simulink model "starmac_system"  (Simulink 7.1)
settings: Solver=ode45  StartTime=0.0  StopTime=30  FixedStep=.001  MaxStep=.01  RelTol=1e-4
undefined symbols (not defined in the file or in its folder): DiscIntNeverNeededParam, ToverTh
libraries: simulink x12, aero_sim_lib x1
settings Model: Creator=Administrator  LastModifiedBy=Administrator

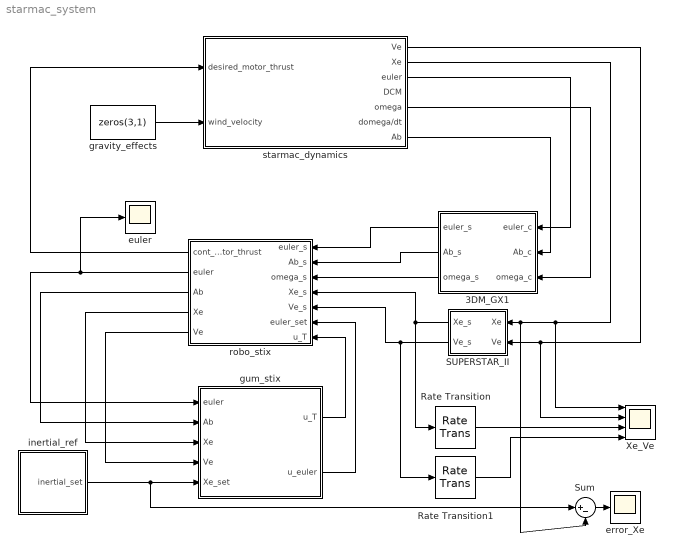
== system starmac_system ==
  3DM_GX1 : Subsystem  Orientation=left  mask{a_g_s=7000, g_max=5, g_g_s=8500, omega_max=300, Ts=.01}
      mask prompts: a_g_s "AccelGainScale:"; g_max "Max G (1 G = 9.81 m/s^2):"; g_g_s "GyroGainScale:"; omega_max "Mav Angular Velocity (deg/sec):"; Ts "Sample Rate (seconds):"
  Rate Transition : RateTransition
  Rate Transition1 : RateTransition
  SUPERSTAR_II : Subsystem  Orientation=left  mask{Ts=.2}
      mask prompts: Ts "Sample Rate (seconds):"
  Sum : Sum  Inputs=|+-  OutDataType=sfix(16)  OutScaling=2^0
  Xe_Ve : Scope  NumInputPorts=4
      settings: YMin=-5~-5~-5~-5  YMax=5~5~5~5
  error_Xe : Scope
      settings: SaveName=ScopeData4
  euler : Scope
  gravity_effects : Constant  Value=zeros(3,1)  OutDataType=sfix(16)  OutScaling=2^0
  gum_stix : Subsystem
  inertial_ref : Subsystem
  robo_stix : Subsystem  Orientation=left
  starmac_dynamics : Subsystem  AncestorBlock=aero_sim_lib/starmac_dynamics  mask{M=1.8263, tau_motor=0.1, b=0.1, select_sub=Select Subsystem}
      mask prompts: M "UAV Mass (kg) [M]:"; tau_motor "Motor Time constant (s)[tau_motor]:"; b "Viscus Drag Coef. (N-s/m)[b]:"; select_sub "Select a model Subsystem:"
      mask StyleString: edit,edit,edit,popup(Select Subsystem|M:starmac_motor_dynamics|B:starmac_blade_flapping_effects|6:6DOF_Euler_Angles)
      mask CallbackString:
      | |||gcb_d=gcb;
      | mask_str = get_param(gcb_d, 'MaskValues');
      | if strcmp(mask_str{4}(1),'M')
      |     open_system([gcb_d '/starmac_motor_dynamics'],'mask');
      | elseif strcmp(mask_str{4}(1),'B')
      |     open_system([gcb_d '/starmac_blade_flapping_effects'],'mask');
      | elseif strcmp(mask_str{4}(1),'6')
      |     open_system([gcb_d '/6DOF_Euler_Angles'],'mask');
      | else
      |     return
      | end
      | set_param(gcb_d,'select_sub','Select Subsystem');
  wires:
  robo_stix/1(cont_motor_thrust) -> starmac_dynamics/1(desired_motor_thrust)
  starmac_dynamics/3(euler) -> 3DM_GX1/1(euler_c)
  starmac_dynamics/7(Ab) -> 3DM_GX1/2(Ab_c)
  starmac_dynamics/5(omega) -> 3DM_GX1/3(omega_c)
  3DM_GX1/1(euler_s) -> robo_stix/1(euler_s)
  3DM_GX1/2(Ab_s) -> robo_stix/2(Ab_s)
  3DM_GX1/3(omega_s) -> robo_stix/3(omega_s)
  robo_stix/2(euler) -> gum_stix/1(euler), euler/1
  robo_stix/4(Xe) -> gum_stix/3(Xe)
  robo_stix/5(Ve) -> gum_stix/4(Ve)
  gum_stix/1(u_T) -> robo_stix/7(u_T)
  gum_stix/2(u_euler) -> robo_stix/6(euler_set)
  robo_stix/3(Ab) -> gum_stix/2(Ab)
  SUPERSTAR_II/1(Xe_s) -> robo_stix/4(Xe_s), Rate Transition/1
  SUPERSTAR_II/2(Ve_s) -> robo_stix/5(Ve_s), Rate Transition1/1
  starmac_dynamics/2(Xe) -> Xe_Ve/1, SUPERSTAR_II/1(Xe), Sum/2
  starmac_dynamics/1(Ve) -> SUPERSTAR_II/2(Ve), Xe_Ve/2
  inertial_ref/1(inertial_set) -> gum_stix/5(Xe_set), Sum/1
  gravity_effects/1 -> starmac_dynamics/2(wind_velocity)
  Sum/1 -> error_Xe/1
  Rate Transition/1 -> Xe_Ve/3
  Rate Transition1/1 -> Xe_Ve/4

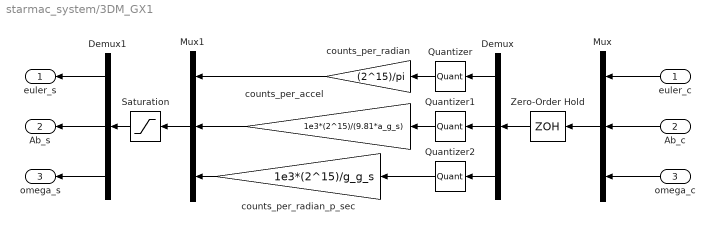
== system starmac_system/3DM_GX1 ==
  euler_c : Inport  Orientation=left
  Ab_c : Inport  Orientation=left  Port=2
  omega_c : Inport  Orientation=left  Port=3
  Demux : Demux  Orientation=left  Outputs=[3 3 3]
  Demux1 : Demux  Orientation=left  Outputs=[3 3 3]
  Mux : Mux  Orientation=left  Inputs=[3 3 3]
  Mux1 : Mux  Orientation=left  Inputs=3
  Quantizer : Quantizer  Orientation=left  QuantizationInterval=pi/(2^15)*ones(3,1)
  Quantizer1 : Quantizer  Orientation=left  QuantizationInterval=g_max*9.81/(2^15)*ones(3,1)
  Quantizer2 : Quantizer  Orientation=left  QuantizationInterval=(pi*omega_max/180)/(2^15)*ones(3,1)
  Saturation : Saturate  Orientation=left  UpperLimit=((2^15)-1)*ones(3*3,1)  LowerLimit=-(2^15)*ones(3*3,1)  OutDataType=sfix(16)  OutScaling=2^0
  Zero-Order Hold : ZeroOrderHold  Orientation=left  SampleTime=Ts
  counts_per_accel : Gain  Orientation=left  Gain=1e3*(2^15)/(9.81*a_g_s)  ParameterDataType=sfix(16)  ParameterScaling=2^0  OutDataType=sfix(16)  OutScaling=2^0
  counts_per_radian : Gain  Orientation=left  Gain=(2^15)/pi  ParameterDataType=sfix(16)  ParameterScaling=2^0  OutDataType=sfix(16)  OutScaling=2^0
  counts_per_radian_p_sec : Gain  Orientation=left  Gain=1e3*(2^15)/g_g_s  ParameterDataType=sfix(16)  ParameterScaling=2^0  OutDataType=sfix(16)  OutScaling=2^0
  euler_s : Outport  Orientation=left
  Ab_s : Outport  Orientation=left  Port=2
  omega_s : Outport  Orientation=left  Port=3
  wires:
  Mux/1 -> Zero-Order Hold/1
  euler_c/1 -> Mux/1
  Ab_c/1 -> Mux/2
  omega_c/1 -> Mux/3
  Zero-Order Hold/1 -> Demux/1
  Demux/1 -> Quantizer/1
  Demux/2 -> Quantizer1/1
  Quantizer/1 -> counts_per_radian/1
  Quantizer1/1 -> counts_per_accel/1
  counts_per_accel/1 -> Mux1/2
  counts_per_radian/1 -> Mux1/1
  Demux/3 -> Quantizer2/1
  counts_per_radian_p_sec/1 -> Mux1/3
  Quantizer2/1 -> counts_per_radian_p_sec/1
  Mux1/1 -> Saturation/1
  Saturation/1 -> Demux1/1
  Demux1/1 -> euler_s/1
  Demux1/2 -> Ab_s/1
  Demux1/3 -> omega_s/1

== system starmac_system/SUPERSTAR_II ==
  Xe : Inport  Orientation=left
  Ve : Inport  Orientation=left  Port=2
  Demux : Demux  Orientation=left  Outputs=[3 3]
  Mux : Mux  Orientation=left  Inputs=[3 3]
  ZOH : ZeroOrderHold  Orientation=left  SampleTime=Ts
  Xe_s : Outport  Orientation=left
  Ve_s : Outport  Orientation=left  Port=2
  wires:
  ZOH/1 -> Demux/1
  Ve/1 -> Mux/2
  Xe/1 -> Mux/1
  Mux/1 -> ZOH/1
  Demux/1 -> Xe_s/1
  Demux/2 -> Ve_s/1

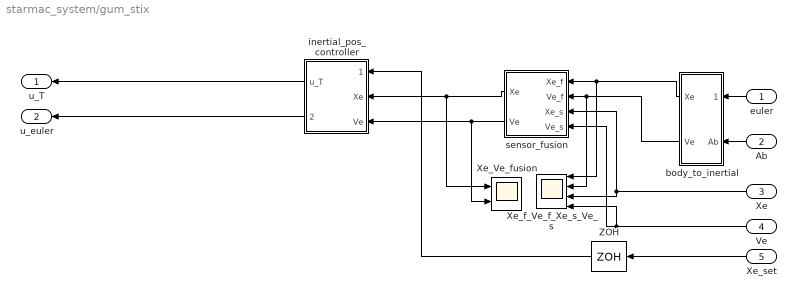
== system starmac_system/gum_stix ==
  euler : Inport  Orientation=left
  Ab : Inport  Orientation=left  Port=2
  Xe : Inport  Orientation=left  Port=3
  Ve : Inport  Orientation=left  Port=4
  Xe_set : Inport  Orientation=left  Port=5
  Xe_Ve_fusion : Scope  NumInputPorts=2
      settings: YMin=-10~-5  YMax=10~5  SaveName=ScopeData2
  Xe_f_Ve_f_Xe_s_Ve_s : Scope  NumInputPorts=4
      settings: YMin=-5~-5~-5~-5  YMax=5~5~5~5  SaveName=ScopeData3
  ZOH : ZeroOrderHold  Orientation=left  SampleTime=.01
  body_to_inertial : Subsystem  Orientation=left
  inertial_pos_controller : Subsystem  Orientation=left  mask{Ts=.01, M=1.8263, K=7.5, K_Ve=2.5}
      mask prompts: Ts "Enter Sample Time [Ts] (seconds):"; M "Enter Mass of UAV [M] (kg):"; K "Enter Loop Gain [K]:"; K_Ve "Enter Velocity Damping Gain [K_Ve]:"
  sensor_fusion : Subsystem  Orientation=left
  u_T : Outport  Orientation=left
  u_euler : Outport  Orientation=left  Port=2
  wires:
  Xe_set/1 -> ZOH/1
  inertial_pos_controller/1(u_T) -> u_T/1
  inertial_pos_controller/2(u_euler) -> u_euler/1
  euler/1 -> body_to_inertial/1(euler)
  Ab/1 -> body_to_inertial/2(Ab)
  sensor_fusion/1(Xe) -> inertial_pos_controller/2(Xe), Xe_Ve_fusion/1
  sensor_fusion/2(Ve) -> inertial_pos_controller/3(Ve), Xe_Ve_fusion/2
  body_to_inertial/1(Xe) -> sensor_fusion/1(Xe_f), Xe_f_Ve_f_Xe_s_Ve_s/1
  body_to_inertial/2(Ve) -> sensor_fusion/2(Ve_f), Xe_f_Ve_f_Xe_s_Ve_s/2
  Xe/1 -> sensor_fusion/3(Xe_s), Xe_f_Ve_f_Xe_s_Ve_s/3
  Ve/1 -> sensor_fusion/4(Ve_s), Xe_f_Ve_f_Xe_s_Ve_s/4
  ZOH/1 -> inertial_pos_controller/1(Xe_set)

== system starmac_system/inertial_ref ==
  Signal Generator : SignalGenerator  Amplitude=20*[1 -1 .5]  Frequency=.5*.0625*ones(3,1)
  inertial_set : Outport
  wires:
  Signal Generator/1 -> inertial_set/1

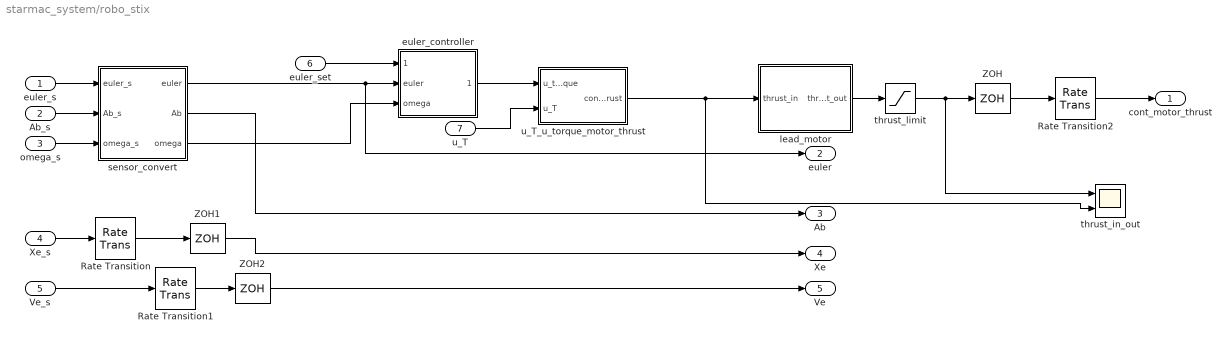
== system starmac_system/robo_stix ==
  euler_s : Inport
  Ab_s : Inport  Port=2
  omega_s : Inport  Port=3
  Xe_s : Inport  Port=4
  Ve_s : Inport  Port=5
  euler_set : Inport  Port=6
  u_T : Inport  Port=7
  Rate Transition : RateTransition
  Rate Transition1 : RateTransition
  Rate Transition2 : RateTransition
  ZOH : ZeroOrderHold  SampleTime=.01
  ZOH1 : ZeroOrderHold  SampleTime=.01
  ZOH2 : ZeroOrderHold  SampleTime=.01
  euler_controller : Subsystem  mask{K=1, K_e=7.5, K_o=.65}
      mask prompts: K "Loop Gain [K]:"; K_e "Euler Gain [K_e]:"; K_o "Omega Gain [K_o]:"
  lead_motor : Subsystem  mask{tau_motor=.1, t_s=.01}
      mask init:
      | a=1/tau_motor;
      | b=pi/t_s;
      | T=t_s;
      | num1=b*(1-exp(-b*T))+a*(b*T-1+exp(-b*T));
      | num2=-b*(1-exp(-b*T))+a*(1-exp(-b*T)-b*T*exp(-b*T));
      | den1=a*b;
      | den2=-a*b*exp(-b*T);
      | num=(b/a)*[num1 num2];
      | den=[den1 den2];
      | Hz=tf(num,den,T);
      | [y,t]=step(Hz);
      | num=(1/y(length(y)))*num;
      | %Hz=(1/y(length(y)))*Hz
      | %bode(Hz);
  sensor_convert : Subsystem  mask{a_g_s=7000, g_g_s=8500}
      mask prompts: a_g_s "AccelGainScale[a_g_s]:"; g_g_s "GyroGainScale[g_g_s]:"
  thrust_in_out : Scope  NumInputPorts=2
      settings: YMin=-5~-5  YMax=5~5  SaveName=ScopeData5
  thrust_limit : Saturate  UpperLimit=10*ones(1,4)  LowerLimit=0*ones(1,4)  OutDataType=sfix(16)  OutScaling=2^0
  u_T_u_torque_motor_thrust : Subsystem  mask{dx=.3048, K_torque=.47}
      mask prompts: dx "X distance of motor from CG [dx](meters):"; K_torque "Ktorque [K_torque]:"
      mask init:
      | M=[0 -dx 0 dx;
      |    dx 0 -dx 0;
      |    -K_torque K_torque -K_torque K_torque;
      |    1 1 1 1];
      | Mi=inv(M);
  cont_motor_thrust : Outport
  euler : Outport  Port=2
  Ab : Outport  Port=3
  Xe : Outport  Port=4
  Ve : Outport  Port=5
  wires:
  euler_s/1 -> sensor_convert/1(euler_s)
  ZOH/1 -> Rate Transition2/1
  Ab_s/1 -> sensor_convert/2(Ab_s)
  omega_s/1 -> sensor_convert/3(omega_s)
  sensor_convert/1(euler) -> euler_controller/2(euler), euler/1
  euler_set/1 -> euler_controller/1(euler_set)
  sensor_convert/3(omega) -> euler_controller/3(omega)
  u_T/1 -> u_T_u_torque_motor_thrust/2(u_T)
  Xe_s/1 -> Rate Transition/1
  Ve_s/1 -> Rate Transition1/1
  euler_controller/1(u_torque) -> u_T_u_torque_motor_thrust/1(u_torque)
  sensor_convert/2(Ab) -> Ab/1
  ZOH1/1 -> Xe/1
  ZOH2/1 -> Ve/1
  Rate Transition/1 -> ZOH1/1
  Rate Transition1/1 -> ZOH2/1
  Rate Transition2/1 -> cont_motor_thrust/1
  u_T_u_torque_motor_thrust/1(cont_motor_thrust) -> lead_motor/1(thrust_in), thrust_in_out/2
  thrust_limit/1 -> ZOH/1, thrust_in_out/1
  lead_motor/1(thrust_out) -> thrust_limit/1

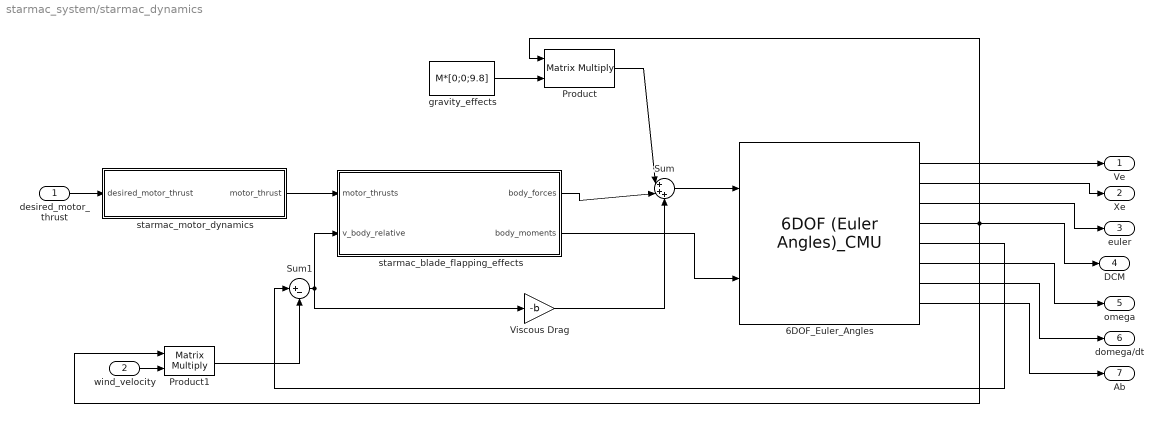
== system starmac_system/starmac_dynamics ==
  desired_motor_thrust : Inport  OutDataType=sfix(16)  OutScaling=2^0
  wind_velocity : Inport  Port=2  OutDataType=sfix(16)  OutScaling=2^0
  6DOF_Euler_Angles : aero_sim_lib/6DOF (Euler Angles)_CMU  SystemSampleTime=-1  XYZe_0=[0.1;0.2;0]  Vb_0=[0;0;0]  euler_0=[0;0;0]  omega_0=[0;0;0]  M=M  I=diag([0.02759 0.02771 0.04806])
  Product : Product  Multiplication=Matrix(*)  OutDataType=sfix(16)  OutScaling=2^0  RndMeth=Zero
  Product1 : Product  Multiplication=Matrix(*)  OutDataType=sfix(16)  OutScaling=2^0  RndMeth=Zero
  Sum : Sum  Inputs=|+++  OutDataType=sfix(16)  OutScaling=2^0
  Sum1 : Sum  Inputs=|+-  OutDataType=sfix(16)  OutScaling=2^0
  Viscous Drag : Gain  Gain=-b  ParameterDataType=sfix(16)  ParameterScaling=2^0  OutDataType=sfix(16)  OutScaling=2^0
  gravity_effects : Constant  Value=M*[0;0;9.8]  OutDataType=sfix(16)  OutScaling=2^0
  starmac_blade_flapping_effects : Subsystem  AncestorBlock=aero_sim_lib/starmac_blade_flapping_effects  mask{select_sub=Select Subsystem}
      mask prompts: select_sub "Select Subsystem:"
      mask help:
      | Allows user to set parameters of various subsystems
      | within the Blade Flapping Effects Model
      mask Help:
      | Select a Subsystem To Set Various
      | Sub System Parameters
      mask StyleString: popup(Select Subsystem|V:starmac_vertical_effect_dynamics|B:starmac_body_moments|F:starmac_flapping_dynamics)
      mask CallbackString:
      | gcb_c=gcb;
      | mask_str = get_param(gcb_c, 'MaskValues');
      | if strcmp(mask_str{1}(1),'V')
      |     open_system([gcb_c '/starmac_vertical_effect_dynamics'],'mask');
      | elseif strcmp(mask_str{1}(1),'B')
      |     open_system([gcb_c '/starmac_body_moments'],'mask');
      | elseif strcmp(mask_str{1}(1),'F')
      |     open_system([gcb_c '/starmac_flapping_dynamics'],'mask');
      | else
      |     return
      | end
      | set_param(gcb_c,'select_sub','Select Subsystem');
  starmac_motor_dynamics : Subsystem  AncestorBlock=aero_sim_lib/starmac_motor_dynamics  mask{tau_motor=tau_motor, T_nom=M*9.8/4, thrust_max=9.8, thrust_min=0, motor_lag_enable=on, motor_variance=(.05*9.8/4)^2, Ts=.01}
      mask prompts: tau_motor "tau_motor (seconds):"; T_nom "nominal thrust (N):"; thrust_max "maximum thrust (N):"; thrust_min "minimum thrust (N):"; motor_lag_enable "Motor Lag Enabled:"; motor_variance "Motor Variance [motor_variance]:"; Ts "Motor Update Rate (seconds):"
  Ve : Outport  OutDataType=sfix(16)  OutScaling=2^0
  Xe : Outport  Port=2  OutDataType=sfix(16)  OutScaling=2^0
  euler : Outport  Port=3  OutDataType=sfix(16)  OutScaling=2^0
  DCM : Outport  Port=4  OutDataType=sfix(16)  OutScaling=2^0
  omega : Outport  Port=5  OutDataType=sfix(16)  OutScaling=2^0
  domega/dt : Outport  Port=6  OutDataType=sfix(16)  OutScaling=2^0
  Ab : Outport  Port=7  OutDataType=sfix(16)  OutScaling=2^0
  wires:
  6DOF_Euler_Angles/8 -> Ab/1
  6DOF_Euler_Angles/7 -> domega/dt/1
  6DOF_Euler_Angles/6 -> omega/1
  6DOF_Euler_Angles/3 -> euler/1
  6DOF_Euler_Angles/2 -> Xe/1
  6DOF_Euler_Angles/1 -> Ve/1
  starmac_motor_dynamics/1(motor_thrust) -> starmac_blade_flapping_effects/1(motor_thrusts)
  Product/1 -> Sum/1
  Sum/1 -> 6DOF_Euler_Angles/1
  6DOF_Euler_Angles/4 -> DCM/1, Product/1, Product1/1
  gravity_effects/1 -> Product/2
  Sum1/1 -> starmac_blade_flapping_effects/2(v_body_relative), Viscous Drag/1
  Product1/1 -> Sum1/2
  6DOF_Euler_Angles/5 -> Sum1/1
  Viscous Drag/1 -> Sum/3
  starmac_blade_flapping_effects/2(body_moments) -> 6DOF_Euler_Angles/2
  starmac_blade_flapping_effects/1(body_forces) -> Sum/2
  desired_motor_thrust/1 -> starmac_motor_dynamics/1(desired_motor_thrust)
  wind_velocity/1 -> Product1/2

== system starmac_system/gum_stix/body_to_inertial ==
  euler : Inport  Orientation=left
  Ab : Inport  Orientation=left  Port=2
  Ab_to_Ae : Stateflow chart  Orientation=left
  Mux : Mux  Orientation=left  Inputs=[3 3]
  inertial_vel_and pos_est : Subsystem  Orientation=left  mask{Ts=.01}
      mask prompts: Ts "Sample Time [Ts] (seconds):"
  Xe : Outport  Orientation=left
  Ve : Outport  Orientation=left  Port=2
  wires:
  euler/1 -> Mux/1
  Ab/1 -> Mux/2
  inertial_vel_and pos_est/2(Xb) -> Xe/1
  Ab_to_Ae/1(y) -> inertial_vel_and pos_est/1(Ab)
  inertial_vel_and pos_est/1(Vb) -> Ve/1
  Mux/1 -> Ab_to_Ae/1(u)

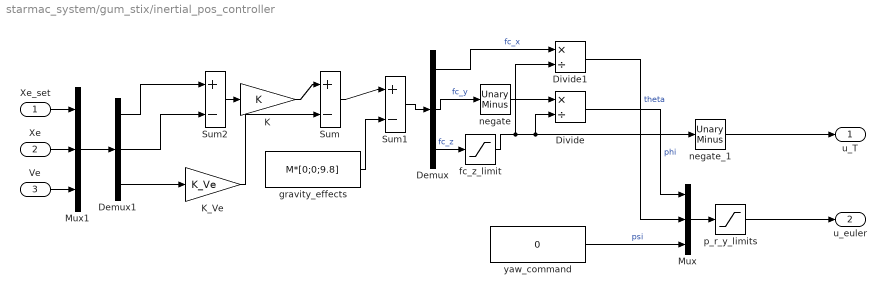
== system starmac_system/gum_stix/inertial_pos_controller ==
  Xe_set : Inport
  Xe : Inport  Port=2
  Ve : Inport  Port=3
  Demux : Demux  Outputs=[1 1 1]
  Demux1 : Demux  Outputs=[3 3 3]
  Divide : Product  Inputs=*/  OutDataType=sfix(16)  OutScaling=2^-10
  Divide1 : Product  Inputs=*/  OutDataType=sfix(16)  OutScaling=2^-10
  K : Gain  Gain=K  ParameterDataType=sfix(16)  ParameterScaling=2^0  OutDataType=sfix(16)  OutScaling=2^0
  K_Ve : Gain  Gain=K_Ve  ParameterDataType=sfix(16)  ParameterScaling=2^0  OutDataType=sfix(16)  OutScaling=2^0
  Mux : Mux  Inputs=[1 1 1]
  Mux1 : Mux  Inputs=[3 3 3]
  Sum : Sum  Inputs=|+-  OutDataType=sfix(16)  OutScaling=2^0
  Sum1 : Sum  Inputs=|+-  OutDataType=sfix(16)  OutScaling=2^0
  Sum2 : Sum  Inputs=|+-  OutDataType=sfix(16)  OutScaling=2^0
  fc_z_limit : Saturate  UpperLimit=-(1/4)*9.81  LowerLimit=-4*9.81  OutDataType=sfix(16)  OutScaling=2^0
  gravity_effects : Constant  Value=M*[0;0;9.8]  OutDataType=sfix(16)  OutScaling=2^0
  negate : simulink/Math Operations/Unary Minus  DoSatur=off
  negate_1 : simulink/Math Operations/Unary Minus  DoSatur=off
  p_r_y_limits : Saturate  UpperLimit=(pi/4)*ones(3,1)  LowerLimit=-(pi/4)*ones(3,1)  OutDataType=sfix(16)  OutScaling=2^0
  yaw_command : Constant  Value=0  OutDataType=sfix(16)  OutScaling=2^0
  u_T : Outport
  u_euler : Outport  Port=2
  wires:
  fc_z_limit/1 -> Divide1/2, negate_1/1, Divide/2
  Demux1/3 -> K_Ve/1
  Mux1/1 -> Demux1/1
  Ve/1 -> Mux1/3
  Xe/1 -> Mux1/2
  Xe_set/1 -> Mux1/1
  K_Ve/1 -> Sum/2
  negate_1/1 -> u_T/1
  p_r_y_limits/1 -> u_euler/1
  Divide1/1 -> Mux/2  "theta"
  Demux/1 -> Divide1/1  "fc_x"
  Divide/1 -> Mux/1  "phi"
  negate/1 -> Divide/1
  Demux/2 -> negate/1  "fc_y"
  yaw_command/1 -> Mux/3  "psi"
  Demux/3 -> fc_z_limit/1  "fc_z"
  Mux/1 -> p_r_y_limits/1
  Sum1/1 -> Demux/1
  gravity_effects/1 -> Sum1/2
  Sum/1 -> Sum1/1
  Demux1/1 -> Sum2/1
  Demux1/2 -> Sum2/2
  Sum2/1 -> K/1
  K/1 -> Sum/1

== system starmac_system/gum_stix/sensor_fusion ==
  Xe_f : Inport  Orientation=left
  Ve_f : Inport  Orientation=left  Port=2
  Xe_s : Inport  Orientation=left  Port=3
  Ve_s : Inport  Orientation=left  Port=4
  Demux : Demux  Orientation=left  Outputs=[3,3]
  Mux : Mux  Orientation=left  Inputs=[3 3 3 3]
  sensor_fusion_fcn : Stateflow chart  Orientation=left
  Xe : Outport  Orientation=left
  Ve : Outport  Orientation=left  Port=2
  wires:
  Mux/1 -> sensor_fusion_fcn/1(u)
  Xe_f/1 -> Mux/1
  Demux/1 -> Xe/1
  Ve_f/1 -> Mux/2
  Demux/2 -> Ve/1
  Xe_s/1 -> Mux/3
  Ve_s/1 -> Mux/4
  sensor_fusion_fcn/1(y) -> Demux/1

== system starmac_system/robo_stix/euler_controller ==
  euler_set : Inport
  euler : Inport  Port=2
  omega : Inport  Port=3
  K : Gain  Gain=K  ParameterDataType=sfix(16)  ParameterScaling=2^0  OutDataType=sfix(16)  OutScaling=2^0
  K_euler : Gain  Gain=K_e  ParameterDataType=sfix(16)  ParameterScaling=2^0  OutDataType=sfix(16)  OutScaling=2^0
  K_omega : Gain  Gain=K_o  ParameterDataType=sfix(16)  ParameterScaling=2^0  OutDataType=sfix(16)  OutScaling=2^0
  Sum : Sum  Inputs=|+-  OutDataType=sfix(16)  OutScaling=2^0
  Sum1 : Sum  Inputs=|+-  OutDataType=sfix(16)  OutScaling=2^0
  torque_limit : Saturate  UpperLimit=9.8*.3048*ones(1,3)  LowerLimit=-9.8*.3048*ones(1,3)  OutDataType=sfix(16)  OutScaling=2^0
  u_torque : Outport
  wires:
  omega/1 -> K_omega/1
  K/1 -> torque_limit/1
  Sum/1 -> K/1
  K_omega/1 -> Sum/2
  euler_set/1 -> Sum1/1
  Sum1/1 -> K_euler/1
  euler/1 -> Sum1/2
  K_euler/1 -> Sum/1
  torque_limit/1 -> u_torque/1

== system starmac_system/robo_stix/lead_motor ==
  thrust_in : Inport
  Demux : Demux
  Mux : Mux
  lead_comp{,1..3} (4 alike) : DiscreteTransferFcn  Numerator=num  Denominator=den  SampleTime=-1
  thrust_out : Outport
  wires:
  thrust_in/1 -> Demux/1
  Mux/1 -> thrust_out/1
  Demux/1 -> lead_comp/1
  lead_comp/1 -> Mux/1
  Demux/2 -> lead_comp1/1
  lead_comp1/1 -> Mux/2
  Demux/3 -> lead_comp2/1
  lead_comp2/1 -> Mux/3
  Demux/4 -> lead_comp3/1
  lead_comp3/1 -> Mux/4

== system starmac_system/robo_stix/sensor_convert ==
  euler_s : Inport
  Ab_s : Inport  Port=2
  omega_s : Inport  Port=3
  accel_per_count : Gain  Gain=(9.81*a_g_s)/(1e3*(2^15))  ParameterDataType=sfix(16)  ParameterScaling=2^0  OutDataType=sfix(16)  OutScaling=2^0
  radian_p_sec_per_count : Gain  Gain=g_g_s/(1e3*(2^15))  ParameterDataType=sfix(16)  ParameterScaling=2^0  OutDataType=sfix(16)  OutScaling=2^0
  radian_per_count : Gain  Gain=pi/(2^15)  ParameterDataType=sfix(16)  ParameterScaling=2^0  OutDataType=sfix(16)  OutScaling=2^0
  euler : Outport
  Ab : Outport  Port=2
  omega : Outport  Port=3
  wires:
  euler_s/1 -> radian_per_count/1
  radian_per_count/1 -> euler/1
  Ab_s/1 -> accel_per_count/1
  accel_per_count/1 -> Ab/1
  omega_s/1 -> radian_p_sec_per_count/1
  radian_p_sec_per_count/1 -> omega/1

== system starmac_system/robo_stix/u_T_u_torque_motor_thrust ==
  u_torque : Inport  Orientation=left
  u_T : Inport  Orientation=left  Port=2
  Gain : Gain  Orientation=left  Gain=Mi  Multiplication=Matrix(K*u)  ParameterDataType=sfix(16)  ParameterScaling=2^0  OutDataType=sfix(16)  OutScaling=2^0
  Mux : Mux  Orientation=left  Inputs=2
  cont_motor_thrust : Outport  Orientation=left
  wires:
  u_torque/1 -> Mux/1
  Mux/1 -> Gain/1
  u_T/1 -> Mux/2
  Gain/1 -> cont_motor_thrust/1

== system starmac_system/starmac_dynamics/starmac_blade_flapping_effects ==
  motor_thrusts : Inport  OutDataType=sfix(16)  OutScaling=2^0
  v_body_relative : Inport  Port=2  OutDataType=sfix(16)  OutScaling=2^0
  Pick First 2 Elements : Constant  Value=[1 0 0; 0 1 0; 0 0 0]  OutDataType=sfix(16)  OutScaling=2^0
  Product : Product  OutDataType=sfix(16)  OutScaling=2^0  RndMeth=Zero
  Product2 : Product  Multiplication=Matrix(*)  OutDataType=sfix(16)  OutScaling=2^0  RndMeth=Zero
  Product4 : Product  OutDataType=sfix(16)  OutScaling=2^0  RndMeth=Zero
  Sum : Sum  Inputs=|++  OutDataType=sfix(16)  OutScaling=2^0
  Sum of Elements : Sum  Inputs=+  OutDataType=sfix(16)  OutScaling=2^-10
  starmac_body_moments : Subsystem  AncestorBlock=aero_sim_lib/starmac_body_moments  mask{dx=.3048, dz=.07, K_torque=.47}
  starmac_flapping_dynamics : Subsystem  AncestorBlock=aero_sim_lib/starmac_flapping_dynamics  mask{K_a1s=.009, K_beta=.23}
  starmac_vertical_effect_dynamics : Subsystem  AncestorBlock=aero_sim_lib/starmac_vertical_effect_dynamics  mask{tau_motor=tau_motor, R=0.127, Alpha=(pi/180)*[-85:5:85], Vinf=[0:0.5:6], Thrust=9.8*[0.3:0.02:0.8]}
      mask prompts: tau_motor "motor time constant (s)"; R "radius of propeller (m)"; Alpha "Alpha (radians)"; Vinf "Vinf (radians)"; Thrust "Propeller Thrust (N)"
      mask init:
      | rho = 1.2;
      | A = pi*R^2;
      | Vh = sqrt(Thrust/(2*rho*A));
      | for i = 1:length(Vh)
      |     for j = 1:length(Vinf)
      |         for k = 1:length(Alpha)
      |             Vi(k,j,i) = find_vi(Vh(i),Vinf(j),Alpha(k));
      |             ToverTh(k,j,i) = min(10,max(0.1,Vh(i)/(Vi(k,j,i)+Vinf(j)*sin(Alpha(k)))));
      |         end
      |     end
      | end
  body_forces : Outport  OutDataType=sfix(16)  OutScaling=2^0
  body_moments : Outport  Port=2  OutDataType=sfix(16)  OutScaling=2^0
  wires:
  starmac_flapping_dynamics/2(rotor_blade_moments) -> Sum/2
  Sum/1 -> body_moments/1
  starmac_body_moments/1(Body Moments) -> Sum/1
  starmac_flapping_dynamics/1(thrust_vector) -> Product4/2, starmac_body_moments/2(Thrust Vector)
  Product4/1 -> body_forces/1
  Sum of Elements/1 -> Product4/1
  Product2/1 -> starmac_flapping_dynamics/1(Vb2_hat)
  v_body_relative/1 -> Product2/2, starmac_vertical_effect_dynamics/2(v_body_relative)
  Pick First 2 Elements/1 -> Product2/1
  motor_thrusts/1 -> Product/1, starmac_vertical_effect_dynamics/1(motor_thrusts)
  starmac_vertical_effect_dynamics/1(thrust_multiplier) -> Product/2
  Product/1 -> Sum of Elements/1, starmac_body_moments/1(Thrust Magnitudes)

== system starmac_system/starmac_dynamics/starmac_motor_dynamics ==
  desired_motor_thrust : Inport  OutDataType=sfix(16)  OutScaling=2^0
  Band-Limited White Noise : simulink/Sources/Band-Limited White Noise  SystemSampleTime=-1  Cov=Ts*motor_variance*ones(4,1)  Ts=Ts  seed=22341+[0 1 2 3]'
  Constant : Constant  Value=motor_lag_enable  OutDataType=sfix(16)  OutScaling=2^0
  Rate Transition : RateTransition
  Saturation : Saturate  UpperLimit=thrust_max*ones(4,1)  LowerLimit=thrust_min*ones(4,1)
  State-Space : StateSpace  A=-(1/tau_motor)*eye(4)  B=(1/tau_motor)*eye(4)  C=eye(4)  D=zeros(4,4)  X0=T_nom*ones(4,1)
  Sum : Sum  Inputs=|++  OutDataType=sfix(16)  OutScaling=2^0
  Switch : Switch  Criteria=u2 > Threshold  OutDataType=sfix(16)  OutScaling=2^0
  motor_thrust : Outport  OutDataType=sfix(16)  OutScaling=2^0
  wires:
  desired_motor_thrust/1 -> State-Space/1, Switch/3
  Sum/1 -> motor_thrust/1
  Saturation/1 -> Sum/1
  Band-Limited White Noise/1 -> Rate Transition/1
  State-Space/1 -> Switch/1
  Switch/1 -> Saturation/1
  Constant/1 -> Switch/2
  Rate Transition/1 -> Sum/2

== system starmac_system/gum_stix/body_to_inertial/inertial_vel_and pos_est ==
  Ab : Inport
  DT_integrator : DiscreteIntegrator  IntegratorMethod=Integration: Trapezoidal  SampleTime=Ts  OutDataType=sfix(16)  OutScaling=2^0  ICPrevOutput=DiscIntNeverNeededParam  ICPrevScaledInput=DiscIntNeverNeededParam
  DT_integrator1 : DiscreteIntegrator  IntegratorMethod=Integration: Trapezoidal  SampleTime=Ts  OutDataType=sfix(16)  OutScaling=2^0  ICPrevOutput=DiscIntNeverNeededParam  ICPrevScaledInput=DiscIntNeverNeededParam
  Vb : Outport
  Xb : Outport  Port=2
  wires:
  DT_integrator/1 -> DT_integrator1/1, Vb/1
  Ab/1 -> DT_integrator/1
  DT_integrator1/1 -> Xb/1

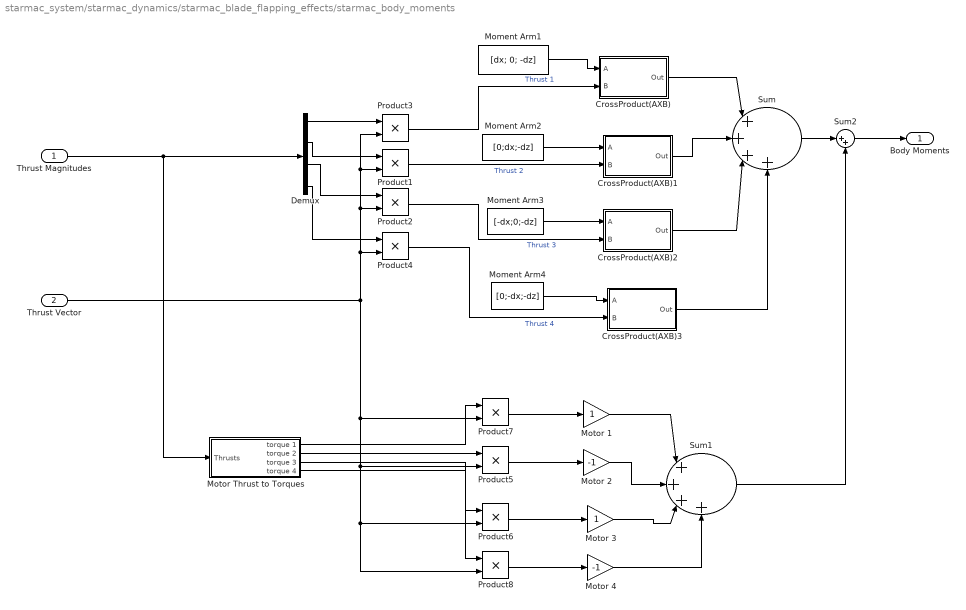
== system starmac_system/starmac_dynamics/starmac_blade_flapping_effects/starmac_body_moments ==
  Thrust Magnitudes : Inport  OutDataType=sfix(16)  OutScaling=2^0
  Thrust Vector : Inport  Port=2  OutDataType=sfix(16)  OutScaling=2^0
  CrossProduct(AXB) : Subsystem
  CrossProduct(AXB)1 : Subsystem
  CrossProduct(AXB)2 : Subsystem
  CrossProduct(AXB)3 : Subsystem
  Demux : Demux
  Moment Arm1 : Constant  Value=[dx; 0; -dz]  OutDataType=sfix(16)  OutScaling=2^0
  Moment Arm2 : Constant  Value=[0;dx;-dz]  OutDataType=sfix(16)  OutScaling=2^0
  Moment Arm3 : Constant  Value=[-dx;0;-dz]  OutDataType=sfix(16)  OutScaling=2^0
  Moment Arm4 : Constant  Value=[0;-dx;-dz]  OutDataType=sfix(16)  OutScaling=2^0
  Motor 1 : Gain  ParameterDataType=sfix(16)  ParameterScaling=2^0  OutDataType=sfix(16)  OutScaling=2^0
  Motor 2 : Gain  Gain=-1  ParameterDataType=sfix(16)  ParameterScaling=2^0  OutDataType=sfix(16)  OutScaling=2^0
  Motor 3 : Gain  ParameterDataType=sfix(16)  ParameterScaling=2^0  OutDataType=sfix(16)  OutScaling=2^0
  Motor 4 : Gain  Gain=-1  ParameterDataType=sfix(16)  ParameterScaling=2^0  OutDataType=sfix(16)  OutScaling=2^0
  Motor Thrust to Torques : Subsystem
  Product{1..8} (8 alike) : Product  OutDataType=sfix(16)  OutScaling=2^0  RndMeth=Zero
  Sum : Sum  Inputs=|++++  OutDataType=sfix(16)  OutScaling=2^0
  Sum1 : Sum  Inputs=|++++  OutDataType=sfix(16)  OutScaling=2^0
  Sum2 : Sum  Inputs=|++  OutDataType=sfix(16)  OutScaling=2^0
  Body Moments : Outport  OutDataType=sfix(16)  OutScaling=2^0
  wires:
  CrossProduct(AXB)1/1(Out) -> Sum/2
  Motor Thrust to Torques/4(torque 4) -> Product8/1
  Motor Thrust to Torques/3(torque 3) -> Product6/1
  Motor Thrust to Torques/2(torque 2) -> Product5/1
  Motor Thrust to Torques/1(torque 1) -> Product7/1
  Product8/1 -> Motor 4/1
  Product6/1 -> Motor 3/1
  Product5/1 -> Motor 2/1
  Product7/1 -> Motor 1/1
  Sum2/1 -> Body Moments/1
  Sum1/1 -> Sum2/2
  Sum/1 -> Sum2/1
  Motor 4/1 -> Sum1/4
  Motor 3/1 -> Sum1/3
  Motor 2/1 -> Sum1/2
  Motor 1/1 -> Sum1/1
  CrossProduct(AXB)3/1(Out) -> Sum/4
  CrossProduct(AXB)2/1(Out) -> Sum/3
  CrossProduct(AXB)/1(Out) -> Sum/1
  Product4/1 -> CrossProduct(AXB)3/2(B)  "Thrust 4"
  Moment Arm4/1 -> CrossProduct(AXB)3/1(A)
  Product2/1 -> CrossProduct(AXB)2/2(B)  "Thrust 3"
  Moment Arm3/1 -> CrossProduct(AXB)2/1(A)
  Product1/1 -> CrossProduct(AXB)1/2(B)  "Thrust 2"
  Moment Arm2/1 -> CrossProduct(AXB)1/1(A)
  Product3/1 -> CrossProduct(AXB)/2(B)  "Thrust 1"
  Moment Arm1/1 -> CrossProduct(AXB)/1(A)
  Thrust Vector/1 -> Product8/2, Product6/2, Product5/2, Product7/2, Product4/2, Product2/2, Product1/2, Product3/2
  Demux/4 -> Product4/1
  Demux/3 -> Product2/1
  Demux/2 -> Product1/1
  Demux/1 -> Product3/1
  Thrust Magnitudes/1 -> Motor Thrust to Torques/1(Thrusts), Demux/1

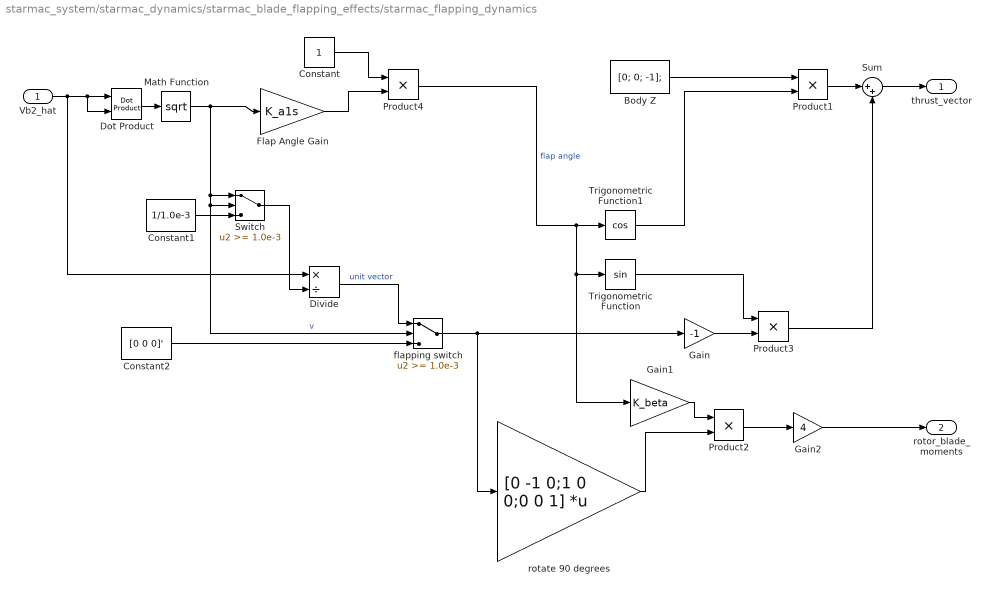
== system starmac_system/starmac_dynamics/starmac_blade_flapping_effects/starmac_flapping_dynamics ==
  Vb2_hat : Inport  OutDataType=sfix(16)  OutScaling=2^0
  "Body Z " : Constant  Value=[0; 0; -1];  OutDataType=sfix(16)  OutScaling=2^0
  Constant : Constant  OutDataType=sfix(16)  OutScaling=2^0
  Constant1 : Constant  Value=1/1.0e-3  OutDataType=sfix(16)  OutScaling=2^0
  Constant2 : Constant  Value=[0 0 0]'  OutDataType=sfix(16)  OutScaling=2^0
  Divide : Product  Inputs=*/  OutDataType=sfix(16)  OutScaling=2^-10
  Dot Product : simulink/Math Operations/Dot Product  InputSameDT=on  OutDataType=sfix(16)  OutScaling=2^-10  DoSatur=off
  Flap Angle Gain : Gain  Gain=K_a1s  ParameterDataType=sfix(16)  ParameterScaling=2^0  OutDataType=sfix(16)  OutScaling=2^0
  Gain : Gain  Gain=-1  ParameterDataType=sfix(16)  ParameterScaling=2^0  OutDataType=sfix(16)  OutScaling=2^0
  Gain1 : Gain  Gain=K_beta  ParameterDataType=sfix(16)  ParameterScaling=2^0  OutDataType=sfix(16)  OutScaling=2^0
  Gain2 : Gain  Gain=4  ParameterDataType=sfix(16)  ParameterScaling=2^0  OutDataType=sfix(16)  OutScaling=2^0
  Math Function : Math  Operator=sqrt  OutDataType=sfix(16)  OutScaling=2^0  SaturateOnIntegerOverflow=on
  Product{1..4} (4 alike) : Product  OutDataType=sfix(16)  OutScaling=2^0  RndMeth=Zero
  Sum : Sum  Inputs=|++  OutDataType=sfix(16)  OutScaling=2^0
  Switch : Switch  Threshold=1.0e-3
  Trigonometric Function : Trigonometry
  Trigonometric Function1 : Trigonometry  Operator=cos
  flapping switch : Switch  Threshold=1.0e-3
  rotate 90 degrees : Gain  Gain=[0 -1 0;1 0 0;0 0 1]  Multiplication=Matrix(K*u)  ParameterDataType=sfix(16)  ParameterScaling=2^0  OutDataType=sfix(16)  OutScaling=2^0
  thrust_vector : Outport  OutDataType=sfix(16)  OutScaling=2^0
  rotor_blade_moments : Outport  Port=2  OutDataType=sfix(16)  OutScaling=2^0
  wires:
  Constant/1 -> Product4/1
  Flap Angle Gain/1 -> Product4/2
  Gain1/1 -> Product2/1
  rotate 90 degrees/1 -> Product2/2
  Product2/1 -> Gain2/1
  Constant2/1 -> flapping switch/3
  flapping switch/1 -> rotate 90 degrees/1, Gain/1
  Divide/1 -> flapping switch/1  "unit vector"
  Constant1/1 -> Switch/3
  Switch/1 -> Divide/2
  Gain2/1 -> rotor_blade_moments/1
  Sum/1 -> thrust_vector/1
  "Body Z "/1 -> Product1/1
  Product1/1 -> Sum/1
  Gain/1 -> Product3/2
  Product3/1 -> Sum/2
  Trigonometric Function/1 -> Product3/1
  Trigonometric Function1/1 -> Product1/2
  Math Function/1 -> Flap Angle Gain/1, flapping switch/2, Switch/2, Switch/1  "v"
  Dot Product/1 -> Math Function/1
  Vb2_hat/1 -> Divide/1, Dot Product/2, Dot Product/1
  Product4/1 -> Gain1/1, Trigonometric Function/1, Trigonometric Function1/1  "flap angle"

== system starmac_system/starmac_dynamics/starmac_blade_flapping_effects/starmac_vertical_effect_dynamics ==
  motor_thrusts : Inport  OutDataType=sfix(16)  OutScaling=2^0
  v_body_relative : Inport  Port=2  OutDataType=sfix(16)  OutScaling=2^0
  Demux : Demux
  Mux : Mux
  starmac_motor_vertical_effect_dynamics : Subsystem  AncestorBlock=aero_sim_lib/starmac_motor_vertical_effect_dynamics  mask{tau_motor=tau_motor, R=R, Alpha=Alpha, Vinf=Vinf, Vh=Vh, ToverTh=ToverTh}
      mask prompts: tau_motor "motor time constant (s)"; R "radius of propeller (m)"; Alpha "Alpha (radians):"; Vinf "Vinf (m/s):"; Vh "Vh (m/s):"
      mask init:
      | rho=1.2;    % kg/m^3, density of air
      | A = pi*R^2; % m^2, area swept out by 1 rotor
  starmac_motor_vertical_effect_dynamics1 : Subsystem  AncestorBlock=aero_sim_lib/starmac_motor_vertical_effect_dynamics  mask{tau_motor=tau_motor, R=R, Alpha=Alpha, Vinf=Vinf, Vh=Vh, ToverTh=ToverTh}
      mask prompts: tau_motor "motor time constant (s)"; R "radius of propeller (m)"; Alpha "Alpha (radians):"; Vinf "Vinf (m/s):"; Vh "Vh (m/s):"
      mask init:
      | rho=1.2;    % kg/m^3, density of air
      | A = pi*R^2; % m^2, area swept out by 1 rotor
  starmac_motor_vertical_effect_dynamics2 : Subsystem  AncestorBlock=aero_sim_lib/starmac_motor_vertical_effect_dynamics  mask{tau_motor=tau_motor, R=R, Alpha=Alpha, Vinf=Vinf, Vh=Vh, ToverTh=ToverTh}
      mask prompts: tau_motor "motor time constant (s)"; R "radius of propeller (m)"; Alpha "Alpha (radians):"; Vinf "Vinf (m/s):"; Vh "Vh (m/s):"
      mask init:
      | rho=1.2;    % kg/m^3, density of air
      | A = pi*R^2; % m^2, area swept out by 1 rotor
  starmac_motor_vertical_effect_dynamics3 : Subsystem  AncestorBlock=aero_sim_lib/starmac_motor_vertical_effect_dynamics  mask{tau_motor=tau_motor, R=R, Alpha=Alpha, Vinf=Vinf, Vh=Vh, ToverTh=ToverTh}
      mask prompts: tau_motor "motor time constant (s)"; R "radius of propeller (m)"; Alpha "Alpha (radians):"; Vinf "Vinf (m/s):"; Vh "Vh (m/s):"
      mask init:
      | rho=1.2;    % kg/m^3, density of air
      | A = pi*R^2; % m^2, area swept out by 1 rotor
  thrust_multiplier : Outport  OutDataType=sfix(16)  OutScaling=2^0
  wires:
  motor_thrusts/1 -> Demux/1
  Mux/1 -> thrust_multiplier/1
  Demux/1 -> starmac_motor_vertical_effect_dynamics/1(motor_thrusts)
  Demux/2 -> starmac_motor_vertical_effect_dynamics1/1(motor_thrusts)
  Demux/3 -> starmac_motor_vertical_effect_dynamics2/1(motor_thrusts)
  Demux/4 -> starmac_motor_vertical_effect_dynamics3/1(motor_thrusts)
  starmac_motor_vertical_effect_dynamics/1(thrust_multiplier) -> Mux/1
  starmac_motor_vertical_effect_dynamics1/1(thrust_multiplier) -> Mux/2
  starmac_motor_vertical_effect_dynamics2/1(thrust_multiplier) -> Mux/3
  starmac_motor_vertical_effect_dynamics3/1(thrust_multiplier) -> Mux/4
  v_body_relative/1 -> starmac_motor_vertical_effect_dynamics2/2(v_body_relative), starmac_motor_vertical_effect_dynamics3/2(v_body_relative), starmac_motor_vertical_effect_dynamics1/2(v_body_relative), starmac_motor_vertical_effect_dynamics/2(v_body_relative)

== system starmac_system/starmac_dynamics/starmac_blade_flapping_effects/starmac_body_moments/CrossProduct(AXB) ==
  A : Inport  OutDataType=sfix(16)  OutScaling=2^0
  B : Inport  Port=2  OutDataType=sfix(16)  OutScaling=2^0
  Fcn : Fcn  Expr=u[2]*u[6]-u[3]*u[5]
  Fcn1 : Fcn  Expr=u[3]*u[4]-u[1]*u[6]
  Fcn2 : Fcn  Expr=u[1]*u[5]-u[2]*u[4]
  Mux : Mux  Inputs=2
  Mux1 : Mux  Inputs=3
  Out : Outport  OutDataType=sfix(16)  OutScaling=2^0
  wires:
  Mux1/1 -> Out/1
  Fcn2/1 -> Mux1/3
  Fcn1/1 -> Mux1/2
  Fcn/1 -> Mux1/1
  Mux/1 -> Fcn2/1, Fcn1/1, Fcn/1
  B/1 -> Mux/2
  A/1 -> Mux/1

== system starmac_system/starmac_dynamics/starmac_blade_flapping_effects/starmac_body_moments/CrossProduct(AXB)1 ==
  A : Inport  OutDataType=sfix(16)  OutScaling=2^0
  B : Inport  Port=2  OutDataType=sfix(16)  OutScaling=2^0
  Fcn : Fcn  Expr=u[2]*u[6]-u[3]*u[5]
  Fcn1 : Fcn  Expr=u[3]*u[4]-u[1]*u[6]
  Fcn2 : Fcn  Expr=u[1]*u[5]-u[2]*u[4]
  Mux : Mux  Inputs=2
  Mux1 : Mux  Inputs=3
  Out : Outport  OutDataType=sfix(16)  OutScaling=2^0
  wires:
  A/1 -> Mux/1
  B/1 -> Mux/2
  Mux/1 -> Fcn/1, Fcn1/1, Fcn2/1
  Fcn/1 -> Mux1/1
  Fcn1/1 -> Mux1/2
  Fcn2/1 -> Mux1/3
  Mux1/1 -> Out/1

== system starmac_system/starmac_dynamics/starmac_blade_flapping_effects/starmac_body_moments/CrossProduct(AXB)2 ==
  A : Inport  OutDataType=sfix(16)  OutScaling=2^0
  B : Inport  Port=2  OutDataType=sfix(16)  OutScaling=2^0
  Fcn : Fcn  Expr=u[2]*u[6]-u[3]*u[5]
  Fcn1 : Fcn  Expr=u[3]*u[4]-u[1]*u[6]
  Fcn2 : Fcn  Expr=u[1]*u[5]-u[2]*u[4]
  Mux : Mux  Inputs=2
  Mux1 : Mux  Inputs=3
  Out : Outport  OutDataType=sfix(16)  OutScaling=2^0
  wires:
  Mux1/1 -> Out/1
  Fcn2/1 -> Mux1/3
  Fcn1/1 -> Mux1/2
  Fcn/1 -> Mux1/1
  Mux/1 -> Fcn2/1, Fcn1/1, Fcn/1
  B/1 -> Mux/2
  A/1 -> Mux/1

== system starmac_system/starmac_dynamics/starmac_blade_flapping_effects/starmac_body_moments/CrossProduct(AXB)3 ==
  A : Inport  OutDataType=sfix(16)  OutScaling=2^0
  B : Inport  Port=2  OutDataType=sfix(16)  OutScaling=2^0
  Fcn : Fcn  Expr=u[2]*u[6]-u[3]*u[5]
  Fcn1 : Fcn  Expr=u[3]*u[4]-u[1]*u[6]
  Fcn2 : Fcn  Expr=u[1]*u[5]-u[2]*u[4]
  Mux : Mux  Inputs=2
  Mux1 : Mux  Inputs=3
  Out : Outport  OutDataType=sfix(16)  OutScaling=2^0
  wires:
  A/1 -> Mux/1
  B/1 -> Mux/2
  Mux/1 -> Fcn/1, Fcn1/1, Fcn2/1
  Fcn/1 -> Mux1/1
  Fcn1/1 -> Mux1/2
  Fcn2/1 -> Mux1/3
  Mux1/1 -> Out/1

== system starmac_system/starmac_dynamics/starmac_blade_flapping_effects/starmac_body_moments/Motor Thrust to Torques ==
  Thrusts : Inport  OutDataType=sfix(16)  OutScaling=2^0
  Demux : Demux
  Gain1 : Gain  Gain=K_torque  ParameterDataType=sfix(16)  ParameterScaling=2^0  OutDataType=sfix(16)  OutScaling=2^0
  torque 1 : Outport  OutDataType=sfix(16)  OutScaling=2^0
  torque 2 : Outport  Port=2  OutDataType=sfix(16)  OutScaling=2^0
  torque 3 : Outport  Port=3  OutDataType=sfix(16)  OutScaling=2^0
  torque 4 : Outport  Port=4  OutDataType=sfix(16)  OutScaling=2^0
  wires:
  Demux/4 -> torque 4/1
  Demux/3 -> torque 3/1
  Demux/2 -> torque 2/1
  Demux/1 -> torque 1/1
  Gain1/1 -> Demux/1
  Thrusts/1 -> Gain1/1

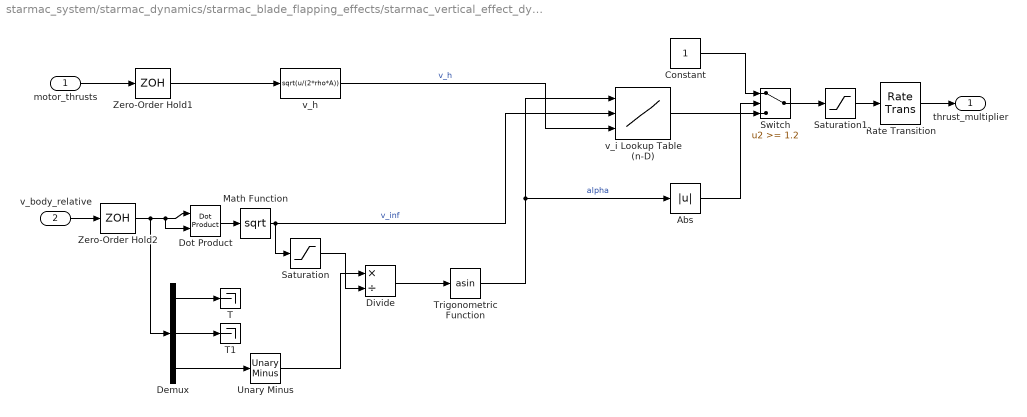
== system starmac_system/starmac_dynamics/starmac_blade_flapping_effects/starmac_vertical_effect_dynamics/starmac_motor_vertical_effect_dynamics ==
  motor_thrusts : Inport  OutDataType=sfix(16)  OutScaling=2^0
  v_body_relative : Inport  Port=2  OutDataType=sfix(16)  OutScaling=2^0
  Abs : Abs
  Constant : Constant  OutDataType=sfix(16)  OutScaling=2^0
  Demux : Demux  Outputs=3
  Divide : Product  Inputs=*/  OutDataType=sfix(16)  OutScaling=2^-10
  Dot Product : simulink/Math Operations/Dot Product  InputSameDT=on  OutDataType=sfix(16)  OutScaling=2^-10  DoSatur=off
  Math Function : Math  Operator=sqrt  OutDataType=sfix(16)  OutScaling=2^0  SaturateOnIntegerOverflow=on
  Rate Transition : RateTransition
  Saturation : Saturate  UpperLimit=500000  LowerLimit=0.0000000001
  Saturation1 : Saturate  UpperLimit=2  LowerLimit=0.5
  Switch : Switch  Threshold=1.2
  T : Terminator
  T1 : Terminator
  Trigonometric Function : Trigonometry  Operator=asin
  Unary Minus : simulink/Math Operations/Unary Minus  DoSatur=off
  Zero-Order Hold1 : ZeroOrderHold  SampleTime=tau_motor
  Zero-Order Hold2 : ZeroOrderHold  SampleTime=tau_motor
  "v_h " : Fcn  Expr=sqrt(u/(2*rho*A))
  v_i Lookup Table (n-D) : Lookup_n-D  NumberOfTableDimensions=3  BreakpointsForDimension1=Alpha  BreakpointsForDimension2=Vinf  BreakpointsForDimension3=Vh  BeginIndexSearchUsingPreviousIndexResult=on  Table=ToverTh  InterpMethod=Cubic spline  InputSameDT=on
  thrust_multiplier : Outport  OutDataType=sfix(16)  OutScaling=2^0
  wires:
  Saturation/1 -> Divide/2
  Demux/3 -> Unary Minus/1
  Unary Minus/1 -> Divide/1
  Abs/1 -> Switch/2
  Constant/1 -> Switch/1
  v_i Lookup Table (n-D)/1 -> Switch/3
  Switch/1 -> Saturation1/1
  Trigonometric Function/1 -> v_i Lookup Table (n-D)/1, Abs/1  "alpha"
  Divide/1 -> Trigonometric Function/1
  Demux/2 -> T1/1
  Demux/1 -> T/1
  Math Function/1 -> Saturation/1, v_i Lookup Table (n-D)/2  "v_inf"
  Dot Product/1 -> Math Function/1
  v_body_relative/1 -> Zero-Order Hold2/1
  motor_thrusts/1 -> Zero-Order Hold1/1
  Zero-Order Hold1/1 -> "v_h "/1
  Zero-Order Hold2/1 -> Demux/1, Dot Product/2, Dot Product/1
  Saturation1/1 -> Rate Transition/1
  "v_h "/1 -> v_i Lookup Table (n-D)/3  "v_h"
  Rate Transition/1 -> thrust_multiplier/1

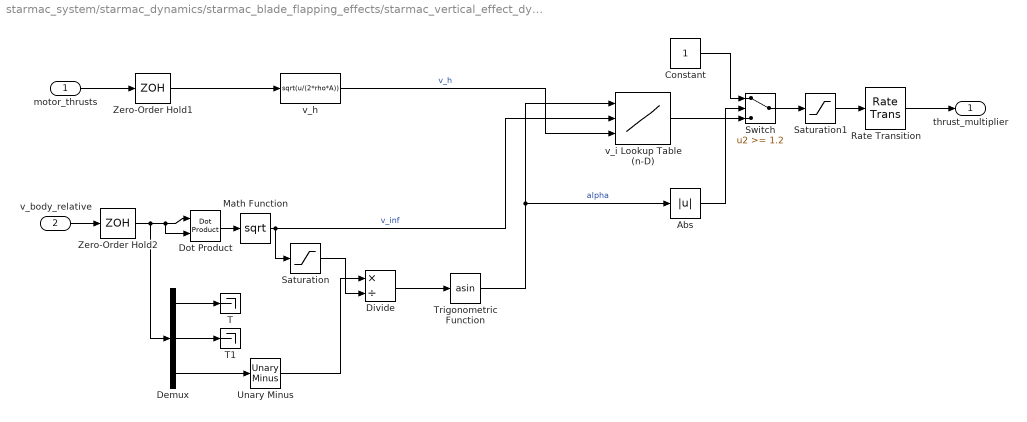
== system starmac_system/starmac_dynamics/starmac_blade_flapping_effects/starmac_vertical_effect_dynamics/starmac_motor_vertical_effect_dynamics1 ==
  motor_thrusts : Inport  OutDataType=sfix(16)  OutScaling=2^0
  v_body_relative : Inport  Port=2  OutDataType=sfix(16)  OutScaling=2^0
  Abs : Abs
  Constant : Constant  OutDataType=sfix(16)  OutScaling=2^0
  Demux : Demux  Outputs=3
  Divide : Product  Inputs=*/  OutDataType=sfix(16)  OutScaling=2^-10
  Dot Product : simulink/Math Operations/Dot Product  InputSameDT=on  OutDataType=sfix(16)  OutScaling=2^-10  DoSatur=off
  Math Function : Math  Operator=sqrt  OutDataType=sfix(16)  OutScaling=2^0  SaturateOnIntegerOverflow=on
  Rate Transition : RateTransition
  Saturation : Saturate  UpperLimit=500000  LowerLimit=0.0000000001
  Saturation1 : Saturate  UpperLimit=2  LowerLimit=0.5
  Switch : Switch  Threshold=1.2
  T : Terminator
  T1 : Terminator
  Trigonometric Function : Trigonometry  Operator=asin
  Unary Minus : simulink/Math Operations/Unary Minus  DoSatur=off
  Zero-Order Hold1 : ZeroOrderHold  SampleTime=tau_motor
  Zero-Order Hold2 : ZeroOrderHold  SampleTime=tau_motor
  "v_h " : Fcn  Expr=sqrt(u/(2*rho*A))
  v_i Lookup Table (n-D) : Lookup_n-D  NumberOfTableDimensions=3  BreakpointsForDimension1=Alpha  BreakpointsForDimension2=Vinf  BreakpointsForDimension3=Vh  BeginIndexSearchUsingPreviousIndexResult=on  Table=ToverTh  InterpMethod=Cubic spline  InputSameDT=on
  thrust_multiplier : Outport  OutDataType=sfix(16)  OutScaling=2^0
  wires:
  Saturation/1 -> Divide/2
  Demux/3 -> Unary Minus/1
  Unary Minus/1 -> Divide/1
  Abs/1 -> Switch/2
  Constant/1 -> Switch/1
  v_i Lookup Table (n-D)/1 -> Switch/3
  Switch/1 -> Saturation1/1
  Trigonometric Function/1 -> v_i Lookup Table (n-D)/1, Abs/1  "alpha"
  Divide/1 -> Trigonometric Function/1
  Demux/2 -> T1/1
  Demux/1 -> T/1
  Math Function/1 -> Saturation/1, v_i Lookup Table (n-D)/2  "v_inf"
  Dot Product/1 -> Math Function/1
  v_body_relative/1 -> Zero-Order Hold2/1
  motor_thrusts/1 -> Zero-Order Hold1/1
  Zero-Order Hold1/1 -> "v_h "/1
  Zero-Order Hold2/1 -> Demux/1, Dot Product/2, Dot Product/1
  Saturation1/1 -> Rate Transition/1
  "v_h "/1 -> v_i Lookup Table (n-D)/3  "v_h"
  Rate Transition/1 -> thrust_multiplier/1

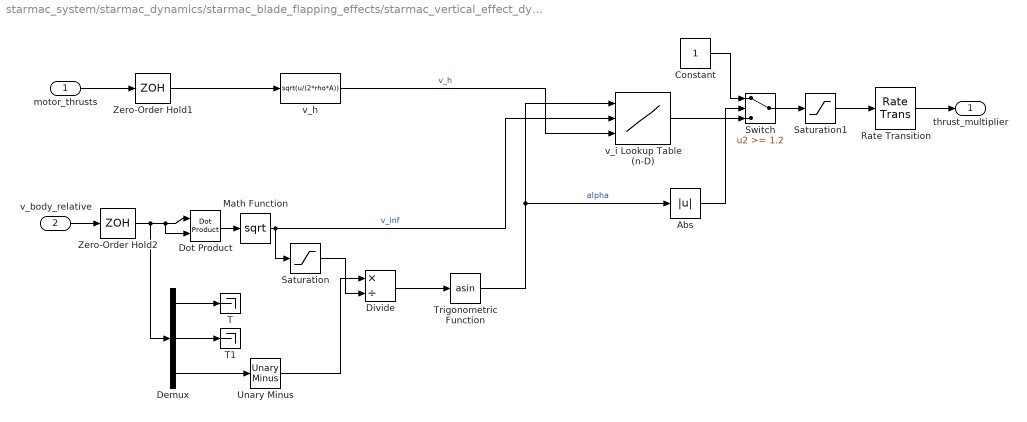
== system starmac_system/starmac_dynamics/starmac_blade_flapping_effects/starmac_vertical_effect_dynamics/starmac_motor_vertical_effect_dynamics2 ==
  motor_thrusts : Inport  OutDataType=sfix(16)  OutScaling=2^0
  v_body_relative : Inport  Port=2  OutDataType=sfix(16)  OutScaling=2^0
  Abs : Abs
  Constant : Constant  OutDataType=sfix(16)  OutScaling=2^0
  Demux : Demux  Outputs=3
  Divide : Product  Inputs=*/  OutDataType=sfix(16)  OutScaling=2^-10
  Dot Product : simulink/Math Operations/Dot Product  InputSameDT=on  OutDataType=sfix(16)  OutScaling=2^-10  DoSatur=off
  Math Function : Math  Operator=sqrt  OutDataType=sfix(16)  OutScaling=2^0  SaturateOnIntegerOverflow=on
  Rate Transition : RateTransition
  Saturation : Saturate  UpperLimit=500000  LowerLimit=0.0000000001
  Saturation1 : Saturate  UpperLimit=2  LowerLimit=0.5
  Switch : Switch  Threshold=1.2
  T : Terminator
  T1 : Terminator
  Trigonometric Function : Trigonometry  Operator=asin
  Unary Minus : simulink/Math Operations/Unary Minus  DoSatur=off
  Zero-Order Hold1 : ZeroOrderHold  SampleTime=tau_motor
  Zero-Order Hold2 : ZeroOrderHold  SampleTime=tau_motor
  "v_h " : Fcn  Expr=sqrt(u/(2*rho*A))
  v_i Lookup Table (n-D) : Lookup_n-D  NumberOfTableDimensions=3  BreakpointsForDimension1=Alpha  BreakpointsForDimension2=Vinf  BreakpointsForDimension3=Vh  BeginIndexSearchUsingPreviousIndexResult=on  Table=ToverTh  InterpMethod=Cubic spline  InputSameDT=on
  thrust_multiplier : Outport  OutDataType=sfix(16)  OutScaling=2^0
  wires:
  Saturation/1 -> Divide/2
  Demux/3 -> Unary Minus/1
  Unary Minus/1 -> Divide/1
  Abs/1 -> Switch/2
  Constant/1 -> Switch/1
  v_i Lookup Table (n-D)/1 -> Switch/3
  Switch/1 -> Saturation1/1
  Trigonometric Function/1 -> v_i Lookup Table (n-D)/1, Abs/1  "alpha"
  Divide/1 -> Trigonometric Function/1
  Demux/2 -> T1/1
  Demux/1 -> T/1
  Math Function/1 -> Saturation/1, v_i Lookup Table (n-D)/2  "v_inf"
  Dot Product/1 -> Math Function/1
  v_body_relative/1 -> Zero-Order Hold2/1
  motor_thrusts/1 -> Zero-Order Hold1/1
  Zero-Order Hold1/1 -> "v_h "/1
  Zero-Order Hold2/1 -> Demux/1, Dot Product/2, Dot Product/1
  Saturation1/1 -> Rate Transition/1
  "v_h "/1 -> v_i Lookup Table (n-D)/3  "v_h"
  Rate Transition/1 -> thrust_multiplier/1

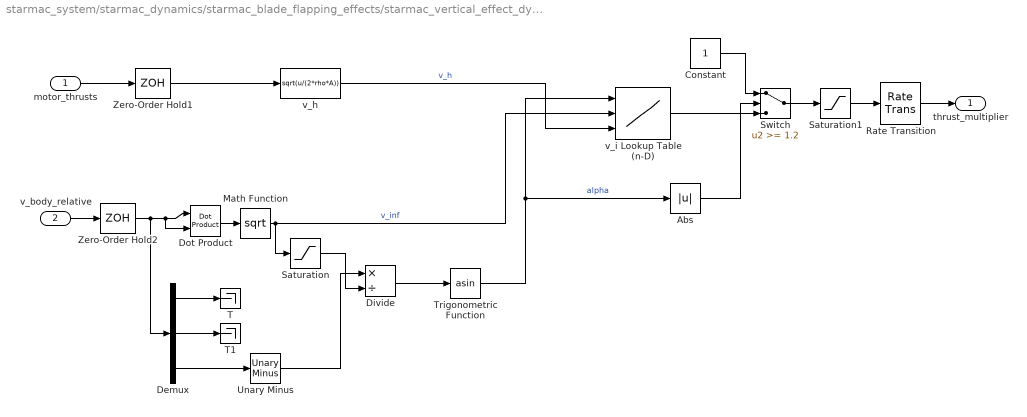
== system starmac_system/starmac_dynamics/starmac_blade_flapping_effects/starmac_vertical_effect_dynamics/starmac_motor_vertical_effect_dynamics3 ==
  motor_thrusts : Inport  OutDataType=sfix(16)  OutScaling=2^0
  v_body_relative : Inport  Port=2  OutDataType=sfix(16)  OutScaling=2^0
  Abs : Abs
  Constant : Constant  OutDataType=sfix(16)  OutScaling=2^0
  Demux : Demux  Outputs=3
  Divide : Product  Inputs=*/  OutDataType=sfix(16)  OutScaling=2^-10
  Dot Product : simulink/Math Operations/Dot Product  InputSameDT=on  OutDataType=sfix(16)  OutScaling=2^-10  DoSatur=off
  Math Function : Math  Operator=sqrt  OutDataType=sfix(16)  OutScaling=2^0  SaturateOnIntegerOverflow=on
  Rate Transition : RateTransition
  Saturation : Saturate  UpperLimit=500000  LowerLimit=0.0000000001
  Saturation1 : Saturate  UpperLimit=2  LowerLimit=0.5
  Switch : Switch  Threshold=1.2
  T : Terminator
  T1 : Terminator
  Trigonometric Function : Trigonometry  Operator=asin
  Unary Minus : simulink/Math Operations/Unary Minus  DoSatur=off
  Zero-Order Hold1 : ZeroOrderHold  SampleTime=tau_motor
  Zero-Order Hold2 : ZeroOrderHold  SampleTime=tau_motor
  "v_h " : Fcn  Expr=sqrt(u/(2*rho*A))
  v_i Lookup Table (n-D) : Lookup_n-D  NumberOfTableDimensions=3  BreakpointsForDimension1=Alpha  BreakpointsForDimension2=Vinf  BreakpointsForDimension3=Vh  BeginIndexSearchUsingPreviousIndexResult=on  Table=ToverTh  InterpMethod=Cubic spline  InputSameDT=on
  thrust_multiplier : Outport  OutDataType=sfix(16)  OutScaling=2^0
  wires:
  Saturation/1 -> Divide/2
  Demux/3 -> Unary Minus/1
  Unary Minus/1 -> Divide/1
  Abs/1 -> Switch/2
  Constant/1 -> Switch/1
  v_i Lookup Table (n-D)/1 -> Switch/3
  Switch/1 -> Saturation1/1
  Trigonometric Function/1 -> v_i Lookup Table (n-D)/1, Abs/1  "alpha"
  Divide/1 -> Trigonometric Function/1
  Demux/2 -> T1/1
  Demux/1 -> T/1
  Math Function/1 -> Saturation/1, v_i Lookup Table (n-D)/2  "v_inf"
  Dot Product/1 -> Math Function/1
  v_body_relative/1 -> Zero-Order Hold2/1
  motor_thrusts/1 -> Zero-Order Hold1/1
  Zero-Order Hold1/1 -> "v_h "/1
  Zero-Order Hold2/1 -> Demux/1, Dot Product/2, Dot Product/1
  Saturation1/1 -> Rate Transition/1
  "v_h "/1 -> v_i Lookup Table (n-D)/3  "v_h"
  Rate Transition/1 -> thrust_multiplier/1

== matlab function gum_stix/body_to_inertial/Ab_to_Ae ==
  data: u input double size=6; y output double
function y = fcn(u)
% This block supports the Embedded MATLAB subset.
% See the help menu for details. 
phi=u(1);
theta=u(2);
psi=u(3);
c_phi=cos(phi);
c_theta=cos(theta);
c_psi=cos(psi);
s_phi=sin(phi);
s_theta=sin(theta);
s_psi=sin(psi);
R=[c_theta*c_psi, c_theta*s_psi, -s_theta;
   s_phi*s_theta*c_psi-c_phi*s_psi, s_phi*s_theta*s_psi+c_phi*c_psi, c_theta*s_phi;
   c_phi*s_theta*c_psi+s_phi*s_psi, c_phi*s_theta*s_psi-s_phi*c_psi, c_theta*c_phi];
Ae= R' * [u(4);u(5);u(6)];
[m,n]=size(u);
if m > n
    y = Ae;
else
    y = Ae';
end

== matlab function gum_stix/sensor_fusion/sensor_fusion_fcn ==
  data: u input double; y output double
function y = fcn(u)
% This block supports the Embedded MATLAB subset.
% See the help menu for details. 
persistent Xe_sh;
persistent dX;
persistent Ve_sh;
persistent dV;
Xe_f = u(1:3);
Ve_f = u(4:6);
Xe_s = u(7:9);
Ve_s = u(10:12);
if isempty(Xe_sh)
    Xe_sh = Xe_s;
    dX = Xe_f - Xe_s;
    Ve_sh = Ve_s;
    dV = Ve_f - Ve_s;
end
if Xe_s(1) ~= Xe_sh(1) || Xe_s(2) ~= Xe_sh(2) || Xe_s(3) ~= Xe_sh(3)
    Xe_sh = Xe_s;
    dX = Xe_f - Xe_s;
end
if Ve_s(1) ~= Ve_sh(1) || Ve_s(2) ~= Ve_sh(2) || Ve_s(3) ~= Ve_sh(3)
    Ve_sh = Ve_s;
    dV = Ve_f - Ve_s;
end
Xe = Xe_f - dX;
Ve = Ve_f - dV;
[m,n] = size(Xe);
if m > n
    y = [Xe;Ve];
else
    y = [Xe,Ve]';
end
